simulink model "decouple"  (R2017a)
settings: Solver=VariableStepAuto  StartTime=0.0  StopTime=20  RelTol=1e-3
values from neighbouring files (symbols this model uses):
  A = [-8.8487+(a-b)/5 -0.0399 -5.55+(c+d)/10 3.5846 ... (first row only)    [initialize.m]
  B = [0.0564+b/(10+c) 0.0319 ... (first row only)    [initialize.m]
  C = [-3.2988 -2.1932+(10*c+d)/(100+5*a) 0.037 -0.0109 ... (first row only)    [initialize.m]
  F = inv(B_star)    [decoupling.m]
  K = q*KT    [MIMO_servo_control_with_observer.m]    (also in decoupling.m = F*C_star_star; full_order_observer.m; pole_placement.m)
settings Model: Creator=lenovo  LastModifiedBy=lenovo

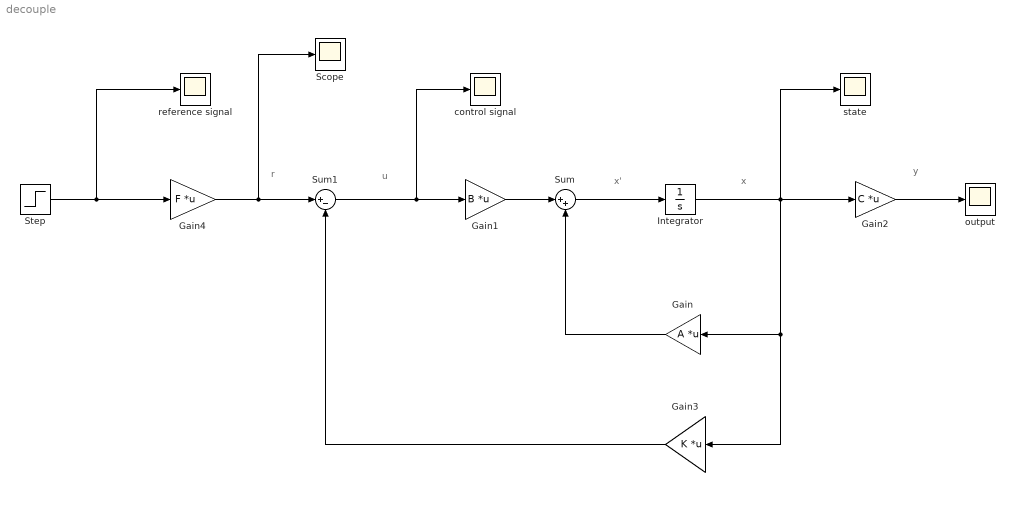
== system decouple ==
  note: u
  note: x
  note: x'
  note: r
  note: y
  Gain : Gain  Gain=A  Multiplication=Matrix(K*u)
  Gain1 : Gain  Gain=B  Multiplication=Matrix(K*u)
  Gain2 : Gain  Gain=C  Multiplication=Matrix(K*u)
  Gain3 : Gain  Gain=K  Multiplication=Matrix(K*u)
  Gain4 : Gain  Gain=F  Multiplication=Matrix(K*u)
  Integrator : Integrator  InitialCondition=[0.5;-0.1;0.3;-0.8]
  Scope : Scope
  Step : Step  Before=[0;0]  After=[1;0]  SampleTime=0  VectorParams1D=off
  Sum : Sum  Inputs=|++
  Sum1 : Sum  Inputs=|+-
  control signal : Scope
  output : Scope
  reference signal : Scope
  state : Scope
  wires:
  Sum/1 -> Integrator/1
  Integrator/1 -> Gain3/1, Gain/1, Gain2/1, state/1
  Sum1/1 -> control signal/1, Gain1/1
  Gain3/1 -> Sum1/2
  Gain1/1 -> Sum/1
  Gain2/1 -> output/1
  Gain/1 -> Sum/2
  Gain4/1 -> Scope/1, Sum1/1
  Step/1 -> reference signal/1, Gain4/1
